simulink library "Lib_Turbo_CompressorVG_TMATS"  (R2015a)
settings: Solver=ode45  StartTime=0.0  StopTime=10.0  RelTol=1e-3
undefined symbols (not defined in the file): stripchar_TMATS
libraries: Lib_Solve_DataOut_TMATS x1
Description:
  | Thomas Modules
settings Model: Creator=jwchapm2  LastModifiedBy=jwchapm2
settings OptimizationCC: ExpressionDepthLimit=2147483647
settings DebuggingCC: UnderspecifiedInitializationDetection=Classic  MergeDetectMultiDrivingBlocksExec=none  SolverPrmCheckMsg=warning  StateNameClashWarn=warning

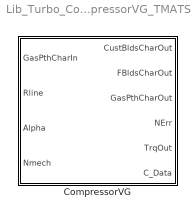
== system Lib_Turbo_CompressorVG_TMATS ==
  CompressorVG : Subsystem  mask(T-MATS: CompressorVG Library Block){X_C_RlineVec_M=[1.0 2.0 3.0], Z_C_AlphaVec_M=[1 2], Y_C_Map_NcVec_M=[0.50 0.80 0.90  1.05], T_C_Map_WcArray_M=ones(4,3,2), T_C_Map_PRArray_M=ones(4,3,2), T_C_Map_EffArray_M=ones(4,3,2), s_C_Nc_M=0.0001, s_C_Wc_M=0.4953, s_C_PR_M=0.8636, s_C_Eff_M=0.9977, SL_M=off, Scale_M=none, CBLDEN_M=off, C_CBD_M=0, C_CBFht_M=0.5, C_CBFPt_M=0.5, FBLDEN_M=off, C_FBD_M=0, C_BFht_M=0.5, C_BFPt_M=0.5, DefSMEn_M=on, SRline_M=1, X_C_Map_WcSurgeVec_M=ones(4,2), T_C_Map_PRSurgeVec_M=ones(4,2), iDesign_M=2, NcDes_M=10000, EffDes_M=0.95, PRDes_M=20, RlineDes_M=2, FVar_M=strcat('iDes_',stripchar_TMATS(gcb),'.bin'), BlkNm_M=double(gcb), HP_M=off}
      mask prompts: X_C_RlineVec_M "X_C_RlineVec_M - Compressor Map Rline Vector (X-axis)(nx1)"; Z_C_AlphaVec_M "Z_C_Map_AlphaVec_M - Compressor Alpha Vector (Z-axis)(rx1)"; Y_C_Map_NcVec_M "Y_C_Map_NcVec_M - Compressor Map Corrected Speed Vector (Y-axis)(mx1)"; T_C_Map_WcArray_M "T_C_Map_WcArray_M - Compressor Map Flow Array (Wc = f(Nc, Rline,Alpha))(mxnxr)"; T_C_Map_PRArray_M "T_C_Map_PRArray_M - Compressor Map Pressure Ratio Array (PR = f(Nc, Rline,Alpha))(mxnxr)"; T_C_Map_EffArray_M "T_C_Map_EffArray_M - Compressor Map Efficiency Array (Eff = f(Nc, Rline,Alpha)(mxnxr)"; s_C_Nc_M "s_C_Nc_M - Corrected Speed Scalar Constant (C_Nc)"; s_C_Wc_M "s_C_Wc_M - Flow Scalar Constant (C_Wc)"; s_C_PR_M "s_C_PR_M - Pressure Ratio Scalar Constant (C_PR)"; s_C_Eff_M "s_C_Eff_M - Efficiency Scalar Constant (C_Eff)"; SL_M "Include surge line"; Scale_M "Scalars"; CBLDEN_M "CBLDEN_M - Customer Bleed Enable [0 - off, 1 - on]"; C_CBD_M "C_CBD_M - Customer or Flow based Bleed Demand[pps] (cbx1)"; C_CBFht_M "C_CBFht_M - Customer or Flow based Bleed Fractional enthalpy[frac] (cbx1)"; C_CBFPt_M "C_CBFPt_M - Customer or Flow based Bleed Fractional Total Pressure[frac] (cbx1)"; FBLDEN_M "FBLDEN_M - Fractional Bleed Enable [0 - off, 1 - on]"; C_FBD_M "C_FBD_M - Fractional Bleed Demand[frac] (bx1)"; C_BFht_M "C_BFht_M - Engine Bleed Fractional Enthalpy[frac] (bx1)"; C_BFPt_M "C_BFPt_M - Engine Bleed Fractional Total Pressure[frac] (bx1)"; DefSMEn_M "DefSMEn_M - Use map default (Rline = 1) surge line"; SRline_M "SRline_M - Rline defined as surge line"; X_C_Map_WcSurgeVec_M "X_C_Map_WcSurgeVec_M - map Compensated flow surge vector (Vec = f(Alpha)) (sxr)"; T_C_Map_PRSurgeVec_M "T_C_Map_PRSurgeVec_M - map Surge Line Pressure Ratio vector (Vec = f(Alpha)) (sxr)"; iDesign_M "iDesign_M - Design fork (0 - Enable iDes, 1 - Use iDes Scalars, 2 - Use Specified Input Scalars)"; NcDes_M "NcDes_M - map Design Corrected Shaft Speed [rpm]"; EffDes_M "EffDes_M  - Design Efficiency [frac]"; PRDes_M "PRDes_M - Design Pressure Ratio [frac]"; RlineDes_M "RlineDes_M - map Design Rline"; FVar_M "FVar_M - File name for iDes Variables"; BlkNm_M "Block name as double for Simulink output"; HP_M "HP_M - Enable Health Parameter input (3x1 vector)"
      mask help:
      | This block simulates the performance of a compressor using basic thermodynamic equations, properties, and table lookups.
      |
      | This block also takes into account 3 dimensional performance maps. Shifting between the tables can be completed using the Alpha term. This feature can be used for simulation of variable geometries.
      mask init:
      | MSK_CompInit_TMATS
      mask Help: web(which('Turbo_TMATS_CmpVG.html'),'-helpbrowser')
      mask TypeOptions Scale_M: none | user defined | iDesign
      mask Callback CBLDEN_M: MSK_SEC_Enables_TMATS('CBLDEN_M',[14 15 16],'en')
      mask Callback FBLDEN_M: MSK_SEC_Enables_TMATS('FBLDEN_M',[18 19 20],'en')
      mask Callback DefSMEn_M:
      | MSK_SEC_Enables_TMATS('DefSMEn_M',[23 24],'dis')
      | MSK_SEC_Enables_TMATS('DefSMEn_M',[22],'en')
      mask Callback iDesign_M:
      | MSK_SEC_Enables_Ides_TMATS('iDesign_M',[7 8 9 10],'G1')
      | MSK_SEC_Enables_Ides_TMATS('iDesign_M',[26 27 28 29],'G2')
      | MSK_SEC_Enables_Ides_TMATS('iDesign_M',[30],'G3')
      mask DialogControl Control2 Prompt: Plot Map
      mask DialogControl Control2 Callback: MSK_PlotCMap_TMATS()

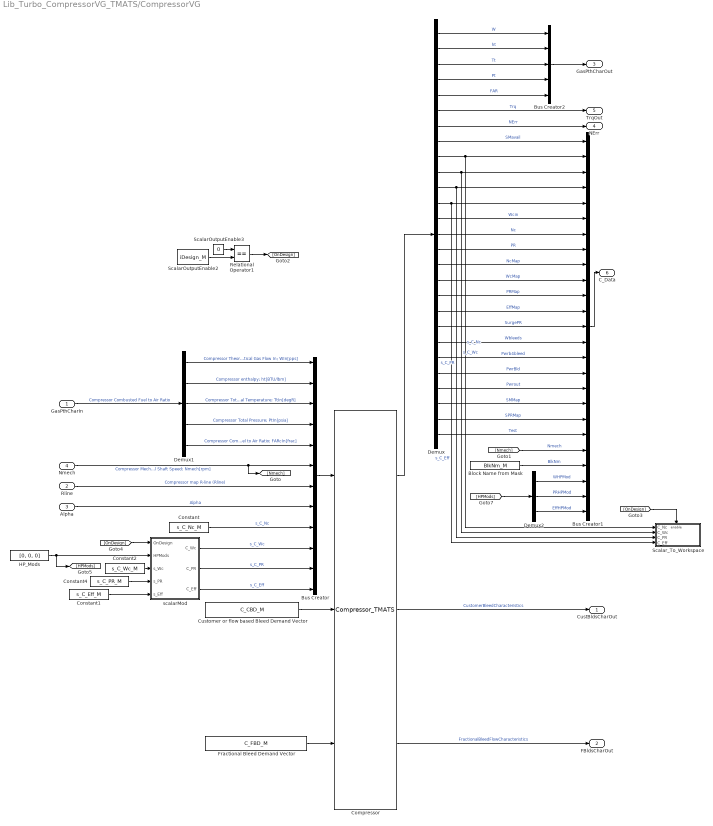
== system Lib_Turbo_CompressorVG_TMATS/CompressorVG ==
  GasPthCharIn : Inport
  Rline : Inport  Port=2
  Alpha : Inport  Port=3
  Nmech : Inport  Port=4
  Block Name from Mask : Constant  Value=BlkNm_M
  Bus Creator : BusCreator  Inputs=12
  Bus Creator1 : BusCreator  Inputs=25
  Bus Creator2 : BusCreator  Inputs=5
  Compressor : S-Function  FunctionName=Compressor_TMATS  Parameters="Y_C_Map_NcVec_M, X_C_RlineVec_M, Z_C_AlphaVec_M, T_C_Map_WcArray_M, T_C_Map_PRArray_M, T_C_Map_EffArray_M, C_CBFht_M, C_CBFPt_M,  C_BFht_M, C_BFPt_M, X_C_Map_WcSurgeVec_M, T_C_Map_PRSurgeVec_M, iDesign_M, NcDes_M, EffDes_M, PRDes_M, RlineDes_M, CBLDEN_M, FBLDEN_M, gcs, length(C_CBD_M), length(C_FBD_M), size(T_C_Map_WcArray_M,2), size(T_C_Map_PRArray_M,2), size(T_C_Map_EffArray_M,2), size(T_C_Map_WcArray_M,1), size(T_C_Map_PRArray_M,1), size(T_C_Map_EffArray_M,1), size(T_C_Map_WcArray_M,3), size(T_C_Map_PRArray_M,3), size(T_C_Map_EffArray_M,3)"  SFunctionModules='h2tc_TMATS pt2sc_TMATS sp2tc_TMATS t2hc_TMATS interp1Ac_TMATS interp2Ac_TMATS interp3Ac_TMATS functions_TMATS'
  Constant : Constant  Value=s_C_Nc_M
  Constant1 : Constant  Value=s_C_Eff_M
  Constant2 : Constant  Value=s_C_Wc_M
  Constant4 : Constant  Value=s_C_PR_M
  Customer or flow based Bleed Demand Vector : Constant  Value=C_CBD_M
  Demux : Demux  Outputs=27
  Demux1 : Demux  Outputs=5
  Demux2 : Demux  Outputs=3
  Fractional Bleed Demand Vector : Constant  Value=C_FBD_M
  HP_Mods : Constant  Value=[0, 0, 0]
  Relational Operator1 : RelationalOperator  Operator===  OutDataTypeStr=boolean
  ScalarOutputEnable2 : Constant  Value=iDesign_M
  ScalarOutputEnable3 : Constant  Value=0
  Scalar_To_Workspace : Subsystem
  scalarMod : Subsystem
  CustBldsCharOut : Outport  PortDimensions=length(C_CBD_M)*5
  FBldsCharOut : Outport  Port=2  PortDimensions=length(C_FBD_M)*5
  GasPthCharOut : Outport  Port=3
  NErr : Outport  Port=4
  TrqOut : Outport  Port=5
  C_Data : Outport  Port=6
  wires:
  Demux1/4 -> Bus Creator/4  "Compressor Total Pressure; PtIn[psia]"
  Nmech/1 -> [Nmech], Bus Creator/6  "Compressor Mechanical Shaft Speed; Nmech[rpm]"
  Demux/6 -> TrqOut/1  "Trq"
  Bus Creator/1 -> Compressor/1
  Demux/4 -> Bus Creator2/4  "Pt"
  Demux/3 -> Bus Creator2/3  "Tt"
  Demux/5 -> Bus Creator2/5  "FAR"
  Demux/1 -> Bus Creator2/1  "W"
  Compressor/1 -> Demux/1
  Demux1/3 -> Bus Creator/3  "Compressor Total Temperature; TtIn[degR]"
  Demux1/5 -> Bus Creator/5  "Compressor Combusted Fuel to Air Ratio; FARcIn[frac]"
  Rline/1 -> Bus Creator/7  "Compressor map R-line (Rline)"
  Demux/13 -> Bus Creator1/6  "Wcin"
  Demux/2 -> Bus Creator2/2  "ht"
  Bus Creator2/1 -> GasPthCharOut/1
  GasPthCharIn/1 -> Demux1/1  "Compressor Combusted Fuel to Air Ratio"
  Demux1/1 -> Bus Creator/1  "Compressor Theoretical Gas Flow In; WIn[pps]"
  Demux/7 -> NErr/1  "NErr"
  Customer or flow based Bleed Demand Vector/1 -> Compressor/2
  Fractional Bleed Demand Vector/1 -> Compressor/3
  Compressor/2 -> CustBldsCharOut/1  "CustomerBleedCharacteristics"
  Compressor/3 -> FBldsCharOut/1  "FractionalBleedFlowCharacteristics"
  Demux1/2 -> Bus Creator/2  "Compressor enthalpy; ht[BTU/lbm]"
  Demux/8 -> Bus Creator1/1  "SMavail"
  Bus Creator1/1 -> C_Data/1
  Demux/9 -> Scalar_To_Workspace/1(C_Nc), Bus Creator1/2  "s_C_Nc"
  Demux/10 -> Scalar_To_Workspace/2(C_Wc), Bus Creator1/3  "s_C_Wc"
  Demux/11 -> Scalar_To_Workspace/3(C_PR), Bus Creator1/4  "s_C_PR"
  Demux/12 -> Scalar_To_Workspace/4(C_Eff), Bus Creator1/5  "s_C_Eff"
  Demux/14 -> Bus Creator1/7  "Nc"
  Demux/23 -> Bus Creator1/16  "PwrBld"
  Demux/22 -> Bus Creator1/15  "Pwrb4bleed"
  Demux/21 -> Bus Creator1/14  "Wbleeds"
  Demux/20 -> Bus Creator1/13  "SurgePR"
  Demux/16 -> Bus Creator1/9  "NcMap"
  Demux/24 -> Bus Creator1/17  "Pwrout"
  Demux/19 -> Bus Creator1/12  "EffMap"
  Demux/17 -> Bus Creator1/10  "WcMap"
  Demux/15 -> Bus Creator1/8  "PR"
  Demux/18 -> Bus Creator1/11  "PRMap"
  Demux/25 -> Bus Creator1/18  "SMMap"
  Demux/26 -> Bus Creator1/19  "SPRMap"
  Demux/27 -> Bus Creator1/20  "Test"
  [Nmech] -> Bus Creator1/21  "Nmech"
  Block Name from Mask/1 -> Bus Creator1/22  "BlkNm"
  scalarMod/3(C_Eff) -> Bus Creator/12  "s_C_Eff"
  scalarMod/1(C_Wc) -> Bus Creator/10  "s_C_Wc"
  scalarMod/2(C_PR) -> Bus Creator/11  "s_C_PR"
  Constant/1 -> Bus Creator/9  "s_C_Nc"
  Alpha/1 -> Bus Creator/8  "Alpha"
  ScalarOutputEnable2/1 -> Relational Operator1/2
  ScalarOutputEnable3/1 -> Relational Operator1/1
  Relational Operator1/1 -> [OnDesign]
  [OnDesign] -> Scalar_To_Workspace/Enable
  Constant2/1 -> scalarMod/3(s_Wc)
  Constant4/1 -> scalarMod/4(s_PR)
  Constant1/1 -> scalarMod/5(s_Eff)
  [OnDesign] -> scalarMod/1(OnDesign)
  HP_Mods/1 -> [HPMods], scalarMod/2(HPMods)
  [HPMods] -> Demux2/1
  Demux2/1 -> Bus Creator1/23  "WHPMod"
  Demux2/2 -> Bus Creator1/24  "PRHPMod"
  Demux2/3 -> Bus Creator1/25  "EffHPMod"

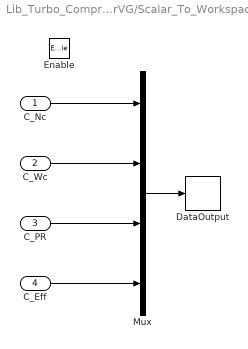
== system Lib_Turbo_CompressorVG_TMATS/CompressorVG/Scalar_To_Workspace ==
  C_Nc : Inport
  C_Wc : Inport  Port=2
  C_PR : Inport  Port=3
  C_Eff : Inport  Port=4
  Enable : EnablePort
  DataOutput : Lib_Solve_DataOut_TMATS/DataOutput  FVar_M=double(FVar_M)
  Mux : Mux
  wires:
  C_Nc/1 -> Mux/1
  C_Wc/1 -> Mux/2
  C_PR/1 -> Mux/3
  C_Eff/1 -> Mux/4
  Mux/1 -> DataOutput/1

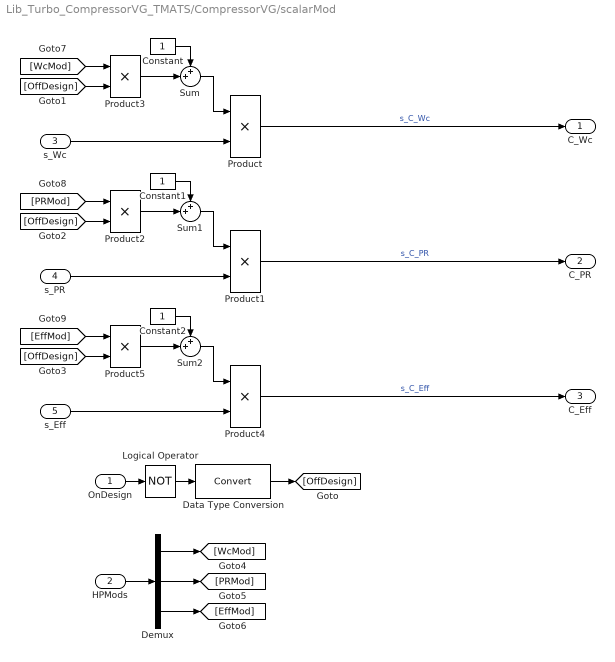
== system Lib_Turbo_CompressorVG_TMATS/CompressorVG/scalarMod ==
  OnDesign : Inport
  HPMods : Inport  Port=2
  s_Wc : Inport  Port=3
  s_PR : Inport  Port=4
  s_Eff : Inport  Port=5
  Constant : Constant
  Constant1 : Constant
  Constant2 : Constant
  Data Type Conversion : DataTypeConversion
  Demux : Demux  Outputs=3
  Logical Operator : Logic  Operator=NOT  AllPortsSameDT=off  OutDataTypeStr=boolean
  Product{,1..5} (6 alike) : Product
  Sum : Sum  Inputs=++|
  Sum1 : Sum  Inputs=++|
  Sum2 : Sum  Inputs=++|
  C_Wc : Outport
  C_PR : Outport  Port=2
  C_Eff : Outport  Port=3
  wires:
  Demux/3 -> [EffMod]
  Demux/2 -> [PRMod]
  Demux/1 -> [WcMod]
  HPMods/1 -> Demux/1
  [OffDesign] -> Product5/2
  Product5/1 -> Sum2/2
  Constant2/1 -> Sum2/1
  [EffMod] -> Product5/1
  Sum2/1 -> Product4/1
  s_Eff/1 -> Product4/2
  [OffDesign] -> Product2/2
  Product2/1 -> Sum1/2
  Constant1/1 -> Sum1/1
  [PRMod] -> Product2/1
  Sum1/1 -> Product1/1
  s_PR/1 -> Product1/2
  [OffDesign] -> Product3/2
  Product3/1 -> Sum/2
  Constant/1 -> Sum/1
  [WcMod] -> Product3/1
  Sum/1 -> Product/1
  Logical Operator/1 -> Data Type Conversion/1
  Data Type Conversion/1 -> [OffDesign]
  OnDesign/1 -> Logical Operator/1
  s_Wc/1 -> Product/2
  Product/1 -> C_Wc/1  "s_C_Wc"
  Product4/1 -> C_Eff/1  "s_C_Eff"
  Product1/1 -> C_PR/1  "s_C_PR"
